simulink model "Triad_activation_libTest"  (R2018b)
settings: Solver=FixedStepDiscrete  StartTime=0.0  StopTime=40  FixedStep=0.1  RelTol=1e-3
undefined symbols (not defined in the file or in its folder): fswParams
libraries: TriadActivation_lib x1
settings Model: Creator=kylle  LastModifiedBy=kylle

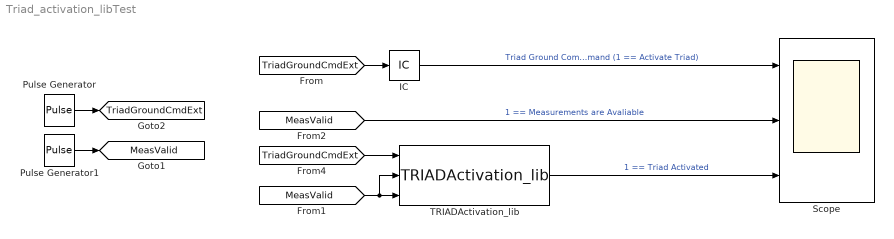
== system Triad_activation_libTest ==
  IC : InitialCondition  Value=fswParams.estimation.ic.activate_triad
  Pulse Generator : DiscretePulseGenerator  PulseType=Time based  Period=10  PhaseDelay=12
  Pulse Generator1 : DiscretePulseGenerator  PulseType=Time based  Period=7  PulseWidth=50  PhaseDelay=3
  Scope : Scope  NumInputPorts=3
  TRIADActivation_lib : TriadActivation_lib/TRIADActivation_lib  SystemSampleTime=-1
  tag scope: MeasValid=global, TriadGroundCmdExt=global
  wires:
  TRIADActivation_lib/1 -> Scope/3  "1 == Triad Activated"
  [MeasValid] -> Scope/2  "1 == Measurements are Avaliable"
  IC/1 -> Scope/1  "Triad Ground Command (1 == Activate Triad)"
  Pulse Generator/1 -> [TriadGroundCmdExt]
  [TriadGroundCmdExt] -> IC/1
  [MeasValid] -> TRIADActivation_lib/2, TRIADActivation_lib/3
  [TriadGroundCmdExt] -> TRIADActivation_lib/1
  Pulse Generator1/1 -> [MeasValid]
